simulink model "Flightsim_aircraft_joystick"  (R2025a)
settings: Solver=FixedStepAuto  StartTime=0.0  StopTime=2000  FixedStep=1/60  MaxStep=0.005  MinStep=0.005  RelTol=1e-6  AbsTol=1e-8
values from neighbouring files (symbols this model uses):
  f = fn{i}    [LandingAnalysis.m]    (also in PerformanceAnalysis.m = @(a) obj.lift_residual(alt, V, M, rho, L_target, a, throttle; TakeoffAnalysis.m)
libraries: simulink_extras x5, instrumentlib x3, aerolibfltsims x2, aerolibobsolete x1, aerolibanimutils x1
settings Model: Creator=naman  LastModifiedBy=namanshetty29
settings DataIOCC: OutputSaveName=out

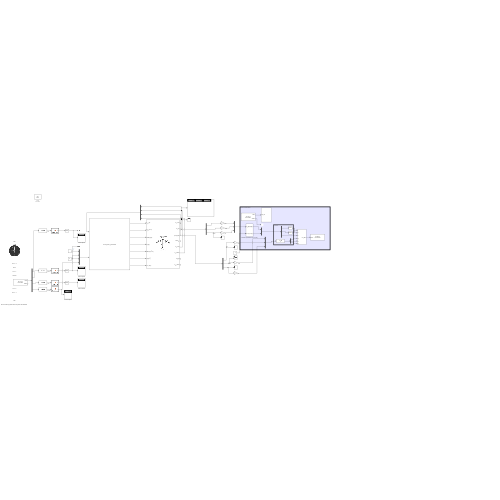
[thumbnail: Simulink's stored preview of the top-level diagram]
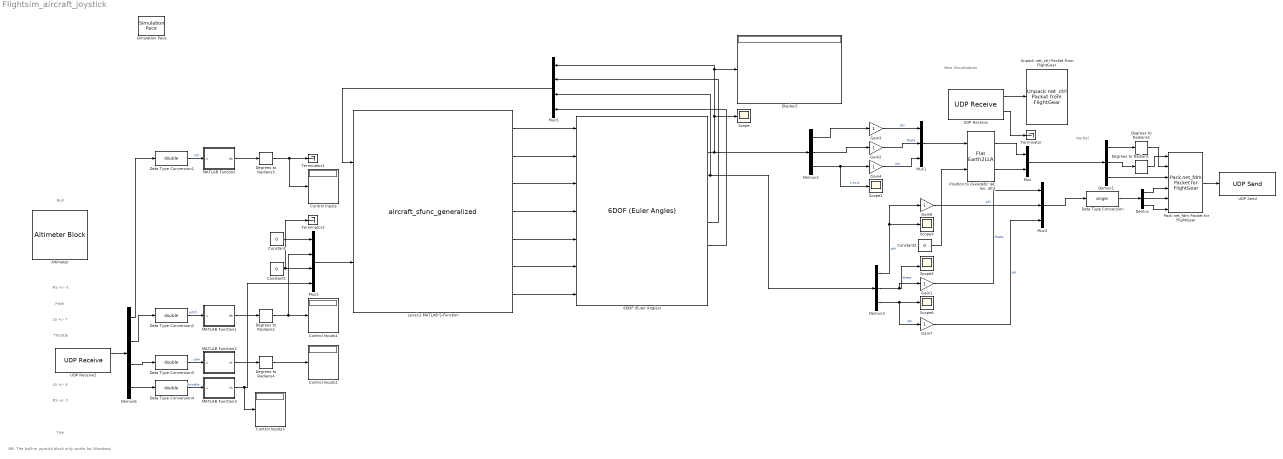
== system Flightsim_aircraft_joystick ==
  note: New Visualization
  note: Inertial
  note: LS +/- Y
  note: RS +/- X
  note: NB: The built-in joystick block only works for Windows!
  note: RS +/- Y
  note: Pitch
  note: Throttle
  note: Roll
  note: LS +/- X
  note: Yaw
  6DOF (Euler Angles) : aerolibobsolete/6DOF (Euler Angles)  units=Metric (MKS)  mtype=Custom Variable  rep=Euler Angles  xme_0=Initialpos  Vm_0=InitialVel  eul_0=InitialOri  pm_0=InitialRot  mass_0=mass  mass_e=0.5  mass_f=2.0  inertia=Inertia  inertia_e=eye(3)  inertia_f=2*eye(3)  k_quat=1.0  vre_flag=on  abi_flag=off  aMode=0  xme_statename=''  Vm_statename=''  eul_statename=''  quat_statename=''  pm_statename=''  mass_statename=''
  Altimeter : AltimeterBlock
  Constant : Constant  Value=0
  Constant1 : Constant  Value=0
  Constant2 : Constant  Value=0
  Control Inputs{,1..3} (4 alike) : Display
  Data Type Conversion : DataTypeConversion  OutDataTypeStr=single  SaturateOnIntegerOverflow=off  RndMeth=Floor
  Data Type Conversion{1..4} (4 alike) : DataTypeConversion  OutDataTypeStr=double  SaturateOnIntegerOverflow=off  RndMeth=Floor
  Degrees to Radians{,1..4} (5 alike) : simulink_extras/Transformations/Degrees to Radians
  Demux{,1..3} (4 alike) : Demux  Outputs=3
  Demux6 : Demux
  Display5 : Display
  Gain{1..4,6..7} (6 alike) : Gain
  Level-2 MATLAB S-Function : M-S-Function  FunctionName=aircraft_sfunc_generalized
  MATLAB Function : MATLAB Function  TreatAsAtomicUnit=on
  MATLAB Function1 : MATLAB Function  TreatAsAtomicUnit=on
  MATLAB Function2 : MATLAB Function  TreatAsAtomicUnit=on
  MATLAB Function3 : MATLAB Function  TreatAsAtomicUnit=on
  Mux : Mux  Inputs=2
  Mux1 : Mux  Inputs=3
  Mux2 : Mux
  Mux3 : Mux  Inputs=3
  Mux5 : Mux
  Pack net_fdm Packet for FlightGear : aerolibfltsims/Pack net_fdm Packet for FlightGear  FlightGearVersion=v2019.1  ShowPositionAttitudeInputs=on  ShowVelocityAccelerationInputs=off  ShowControlSurfacePositionInputs=off  ShowEngineFuelInputs=off  ShowLandingGearInputs=off  ShowEnvironmentInputs=off  SampleTime=-1  packetVersion=24
  "Position to [Geodetic lat, lon, alti]" : FlatEarth2LLA  R=6378137  LL0=[37.210265015306916, -80.41446644179189]
  Scope{,1,4,6} (4 alike) : Scope
      Scope settings: ActiveDisplayYMinimum=-24027.59886  ActiveDisplayYMaximum=124598.21102
      Scope1 settings: ActiveDisplayYMinimum=-9374.19551853851  ActiveDisplayYMaximum=1041.577279837612
      Scope4 settings: ActiveDisplayYMinimum=-1  ActiveDisplayYMaximum=1
      Scope6 settings: ActiveDisplayYMinimum=-1  ActiveDisplayYMaximum=1  DataLoggingVariableName=ScopeData3
  Scope5 : Scope  NumInputPorts=2
      settings: ActiveDisplayYMinimum=-0.19501577484868554  ActiveDisplayYMaximum=0.36789090497858135  DataLoggingVariableName=ScopeData2
  Simulation Pace : aerolibanimutils/Simulation Pace  SimulationPace=1  SleepMode=Auto  OutputPaceError=off  SampleTime=1/30
  Terminator : Terminator
  Terminator1 : Terminator
  Terminator2 : Terminator
  UDP Receive : instrumentlib/UDP Receive  LocalAddress=127.0.0.1  LocalPort=50001  EnablePortSharing=off  Host=localhost  Port=65343  GetLatestData=on  DataSize=[ 1, 744 ]  DataType=uint8  ASCIIFormatting=%f,  Terminator=LF  CustomTerminator=10  ByteOrder=little-endian  EnableBlockingMode=off  Timeout=10  SampleTime=0.2  SimulateUsing=Interpreted execution
  UDP Receive1 : instrumentlib/UDP Receive  LocalAddress=127.0.0.1  LocalPort=5505  EnablePortSharing=off  Host=localhost  Port=9090  GetLatestData=on  DataSize=[ 1, 4]  DataType=single  ASCIIFormatting=%f,  Terminator=LF  CustomTerminator=10  ByteOrder=little-endian  EnableBlockingMode=off  Timeout=10  SampleTime=1/60  SimulateUsing=Interpreted execution
  UDP Send : instrumentlib/UDP Send  Host=localhost  Port=50000  LocalAddress=127.0.0.1  LocalPort=-1  EnablePortSharing=on  OutputDatagramPacketSize=4096  ByteOrder=big-endian  EnableBlockingMode=on  SimulateUsing=Interpreted execution
  Unpack net_ctrl Packet from FlightGear : aerolibfltsims/Unpack net_ctrl Packet from FlightGear  FlightGearVersion=v2019.1  ShowControlSurfacePositionOutputs=off  ShowEngineFuelOutputs=off  ShowLandingGearOutputs=off  ShowAvionicOutputs=off  ShowEnvironmentOutputs=off  SampleTime=-1  packetVersion=27
  wires:
  Data Type Conversion4/1 -> MATLAB Function3/1(u)  "throttle"
  Demux3/1 -> Gain6/1, Scope4/1  "phi"
  Data Type Conversion3/1 -> MATLAB Function2/1(u)  "yaw"
  Data Type Conversion2/1 -> MATLAB Function1/1(u)  "pitch"
  UDP Receive/1 -> Unpack net_ctrl Packet from FlightGear/1
  MATLAB Function/1(da) -> Degrees to Radians3/1
  Gain4/1 -> Mux1/3  "psi"
  Demux6/4 -> Data Type Conversion4/1
  Demux6/2 -> Data Type Conversion2/1
  Constant/1 -> Mux2/1
  UDP Receive1/1 -> Demux6/1
  Pack net_fdm Packet for FlightGear/1 -> UDP Send/1
  Level-2 MATLAB S-Function/7 -> 6DOF (Euler Angles)/7
  Demux1/1 -> Degrees to Radians1/1
  MATLAB Function2/1(dr) -> Degrees to Radians4/1
  Demux6/3 -> Data Type Conversion3/1
  Demux6/1 -> Data Type Conversion1/1
  UDP Receive/2 -> Terminator/1
  MATLAB Function3/1(th) -> Control Inputs3/1, Mux2/4
  Constant1/1 -> Terminator2/1, Mux2/3
  Demux2/2 -> Gain2/1
  MATLAB Function1/1(de) -> Degrees to Radians2/1
  Demux3/2 -> Gain1/1, Scope5/2  "theta"
  Data Type Conversion/1 -> Demux/1
  Degrees to Radians2/1 -> Control Inputs1/1, Mux2/2
  Level-2 MATLAB S-Function/4 -> 6DOF (Euler Angles)/4
  Level-2 MATLAB S-Function/2 -> 6DOF (Euler Angles)/2
  Demux2/3 -> Gain4/1, Scope1/1  "z axis"
  "Position to [Geodetic lat, lon, alti]"/1 -> Mux/1
  Degrees to Radians4/1 -> Control Inputs2/1
  Degrees to Radians3/1 -> Control Inputs/1, Terminator1/1
  Mux2/1 -> Level-2 MATLAB S-Function/2
  Data Type Conversion1/1 -> MATLAB Function/1(u)  "roll"
  Level-2 MATLAB S-Function/1 -> 6DOF (Euler Angles)/1
  6DOF (Euler Angles)/2 -> Display5/1, Mux5/1, Scope/1, Demux2/1
  6DOF (Euler Angles)/5 -> Mux5/2
  Level-2 MATLAB S-Function/5 -> 6DOF (Euler Angles)/5
  Mux5/1 -> Level-2 MATLAB S-Function/1
  "Position to [Geodetic lat, lon, alti]"/2 -> Mux/2
  Level-2 MATLAB S-Function/6 -> 6DOF (Euler Angles)/6
  6DOF (Euler Angles)/3 -> Demux3/1, Mux5/3
  6DOF (Euler Angles)/6 -> Mux5/4
  Demux2/1 -> Gain3/1
  Demux1/2 -> Degrees to Radians/1
  Level-2 MATLAB S-Function/3 -> 6DOF (Euler Angles)/3
  Gain3/1 -> Mux1/1  "phi"
  Gain2/1 -> Mux1/2  "theta"
  Demux3/3 -> Gain7/1, Scope6/1  "psi"
  Gain7/1 -> Mux3/3  "psi"
  Gain1/1 -> Mux3/1  "theta"
  Mux/1 -> Demux1/1
  Demux1/3 -> Pack net_fdm Packet for FlightGear/3
  Demux/3 -> Pack net_fdm Packet for FlightGear/6
  Gain6/1 -> Mux3/2  "phi"
  Degrees to Radians1/1 -> Pack net_fdm Packet for FlightGear/2
  Degrees to Radians/1 -> Pack net_fdm Packet for FlightGear/1
  Demux/2 -> Pack net_fdm Packet for FlightGear/5
  Demux/1 -> Pack net_fdm Packet for FlightGear/4
  Mux1/1 -> "Position to [Geodetic lat, lon, alti]"/1
  Mux3/1 -> Data Type Conversion/1
  Constant2/1 -> "Position to [Geodetic lat, lon, alti]"/2

== matlab function Flightsim_aircraft_joystick/MATLAB Function ==
  data: u input; da output
function da = aileronmap(u)

u=min(max(u,-1),1);
if u>=0
    da=20*u;
else
    da=20*u;
end
end

== matlab function Flightsim_aircraft_joystick/MATLAB Function2 ==
  data: u input; dr output
function dr =ruddermap(u)

u=min(max(u,-1),1);
if u<=0
    dr=-30*u;
else
    dr=-30*u;
end
end

== matlab function Flightsim_aircraft_joystick/MATLAB Function3 ==
  data: u input; th output
function th =throttlemap(u)

th=min(max(u,0),1);

end

== matlab function Flightsim_aircraft_joystick/MATLAB Function1 ==
  data: u input; de output
function de = elevatormap(u)

u=min(max(u,-1),1);
if u<=0
    de=-25*u;
else
    de=-25*u;
end
end
